simulink model "UltraMaxProPlus"  (R2021a)
settings: Solver=VariableStepAuto  StartTime=0.0  StopTime=2  RelTol=1e-3
undefined symbols (not defined in the file): Ion, Lithium
libraries: spsVoltageMeasurementLib x10, spsCurrentMeasurementLib x8, spsDiodeLib x8, spsSeriesRLCBranchLib x8, spsMeanLib x4, spsMosfetLib x4, spsPowerLib x2, spspowerguiLib x2, spsACVoltageSourceLib x1, spsBatteryLib x1, spsMutualInductanceLib x1, simulink x1
settings Model: SimulationMode=accelerator  Creator=Nishith  LastModifiedBy=Nishith
settings SolverCC: AlgebraicLoopSolver=TrustRegion
settings DebuggingCC: UnconnectedInputMsg=none  UnconnectedOutputMsg=none  UnconnectedLineMsg=none  ArithmeticOperatorsInVariantConditions=warning
settings SFSimCC: CustomCodeUndefinedFunction=UseInterfaceOnly

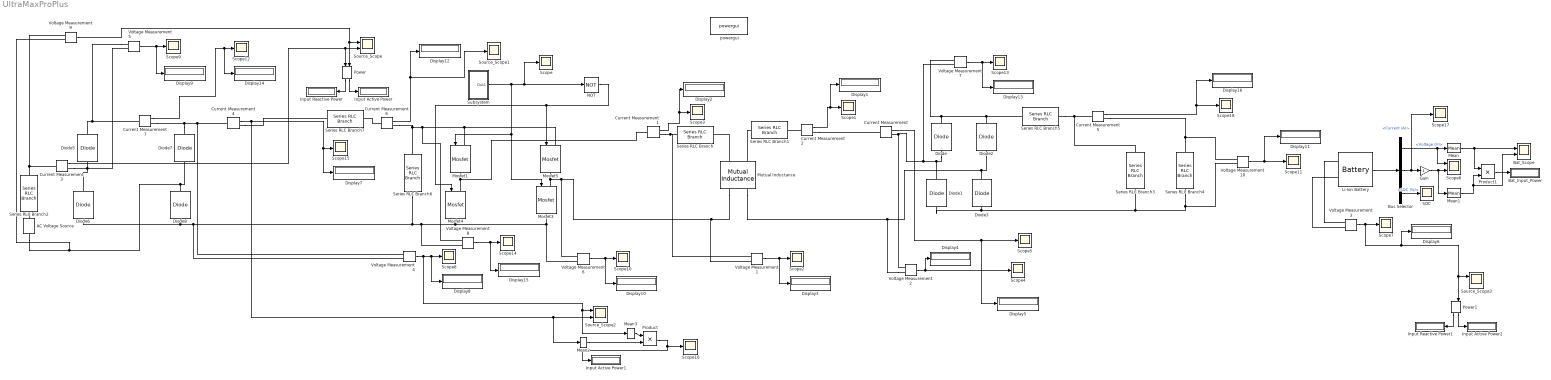
== system UltraMaxProPlus ==
  AC Voltage Source : spsACVoltageSourceLib/AC Voltage Source  Amplitude=325  Phase=0  Frequency=50  SampleTime=0  Measurements=None  BusType=swing  Pref=10e3  Qref=0  Qmin=-inf  Qmax=+inf
  Bat_Input_Power : Display
  Bat_Scope : Scope  NumInputPorts=2
  Bus Selector : BusSelector  OutputSignals=Voltage (V),Current (A),SOC (%)
  Current Measurement{,1..7} (8 alike) : spsCurrentMeasurementLib/Current Measurement  PhasorSimulation=off  OutputType=Complex  PSBequivalent=0
  Diode{,1..3,5..8} (8 alike) : spsDiodeLib/Diode  Ron=0.001  Lon=0  Vf=0.8  IC=0  UseSnubber=0  Rs=500  Cs=250e-9  Measurements=off
  Display{1..16} (16 alike) : Display
  Gain : Gain  Gain=-1
  Input Active Power : Display
  Input Active Power1 : Display
  Input Active Power2 : Display
  Input Reactive Power : Display
  Input Reactive Power1 : Display
  Li-Ion Battery : spsBatteryLib/Battery  BatType=Lithium-Ion  ShowTempParam=off  ThermalPreset=no  ShowAgeParam=off  NomV=120  NomQ=30  SOC=50  Batt_Tr=1  PresetModel=on  MaxQ=30  MinV=90  FullV=139.6785  Dis_rate=13.0435  R=0.04  Normal_OP=27.1304  expZone="[129.6463      1.473913]"  current=[6.5 13 32.5]  Units=Time  Tci=20  NomT=20  T2=-30  MaxQ2=4.8  FullV2=7.1  Normal_OP2=5.655  expZone2="[6.58           1]"  Rca=0.6  ti=2000  Dp=0  Neq0=0  Tsim=1e6  Ta1=25  Qeol=5.4*0.9  Reol=0.013333*1.2  Char_age=[2.3478, 3]  Dis_age=[2.3478, 10]  N1=1500  N2=10500  N3=1000  N4=1400  Ta2=45  N5=950
  Mean : spsMeanLib/Mean  Freq=50  Vinit=0  Ts=0
  Mean1 : spsMeanLib/Mean  Freq=50  Vinit=0  Ts=0
  Mean2 : spsMeanLib/Mean  Freq=60  Vinit=0  Ts=0
  Mean3 : spsMeanLib/Mean  Freq=60  Vinit=0  Ts=0
  Mosfet{1,3..5} (4 alike) : spsMosfetLib/Mosfet  Ron=0.1  Lon=0  Rd=0.01  Vfd=0  IC=0  Rs=1e5  Cs=inf  Measurements=off
  Mutual Inductance : spsMutualInductanceLib/Mutual Inductance  LConnTagsString=a|b  RConnTagsString=A|B  TypeOfMutual=Two or three windings with equal mutual terms  NumberOfWindings=3  SelfImpedance1=[0.001 996.44e-06]  SelfImpedance2=[0.001 107.85e-06]  ThreeWindings=off  SelfImpedance3=[ 1.1 1.1e-03]  MutualImpedance=[0.002 65.5649e-06]  InductanceMatrix="[1.0 0.9  0.9 ;  0.9 1.0  0.9;  0.9 0.9 1.0 ] * 1e-3"  ResistanceMatrix="[1.0 0.9  0.9 ;  0.9 1.0  0.9;  0.9 0.9 1.0 ]"  Measurements=Winding voltages and currents
      settings: SourceProductBaseCode=PS
  NOT : Logic  Operator=NOT  IconShape=distinctive  AllPortsSameDT=off  OutDataTypeStr=boolean
  Power : spsPowerLib/Power  Freq=50  Vinit=[1, 0]  Iinit=[1, 0]  Ts=0
      settings: SourceProductBaseCode=PS
  Power1 : spsPowerLib/Power  Freq=50  Vinit=[1, 0]  Iinit=[1, 0]  Ts=0
      settings: SourceProductBaseCode=PS
  Product : Product
  Product1 : Product
  SOC : Scope
  Scope{,1..5,7..18} (18 alike) : Scope
  Scope6 : Scope  NumInputPorts=2
  Series RLC Branch : spsSeriesRLCBranchLib/Series RLC Branch  LConnTagsString=__new0  RConnTagsString=__new0  BranchType=C  Resistance=1  Inductance=1e-3  SetiL0=off  InitialCurrent=0  Capacitance=3.5184e-9  Setx0=off  InitialVoltage=0  Measurements=None
  Series RLC Branch1 : spsSeriesRLCBranchLib/Series RLC Branch  LConnTagsString=__new0  RConnTagsString=__new0  BranchType=C  Resistance=1  Inductance=1e-3  SetiL0=off  InitialCurrent=0  Capacitance=32.507e-9  Setx0=off  InitialVoltage=0  Measurements=None
  Series RLC Branch2 : spsSeriesRLCBranchLib/Series RLC Branch  LConnTagsString=__new0  RConnTagsString=__new0  BranchType=RL  Resistance=0.1  Inductance=3e-3  SetiL0=off  InitialCurrent=0  Capacitance=1e-6  Setx0=off  InitialVoltage=0  Measurements=None
  Series RLC Branch3 : spsSeriesRLCBranchLib/Series RLC Branch  LConnTagsString=__new0  RConnTagsString=__new0  BranchType=C  Resistance=1  Inductance=1e-3  SetiL0=off  InitialCurrent=0  Capacitance=300e-6  Setx0=off  InitialVoltage=0  Measurements=None
  Series RLC Branch4 : spsSeriesRLCBranchLib/Series RLC Branch  LConnTagsString=__new0  RConnTagsString=__new0  BranchType=R  Resistance=28.8  Inductance=1e-3  SetiL0=off  InitialCurrent=0  Capacitance=1e-6  Setx0=off  InitialVoltage=0  Measurements=None
  Series RLC Branch5 : spsSeriesRLCBranchLib/Series RLC Branch  LConnTagsString=__new0  RConnTagsString=__new0  BranchType=L  Resistance=1  Inductance=5e-3  SetiL0=off  InitialCurrent=0  Capacitance=1e-6  Setx0=off  InitialVoltage=0  Measurements=None
  Series RLC Branch6 : spsSeriesRLCBranchLib/Series RLC Branch  LConnTagsString=__new0  RConnTagsString=__new0  BranchType=C  Resistance=1  Inductance=1e-3  SetiL0=off  InitialCurrent=0  Capacitance=500e-6  Setx0=off  InitialVoltage=0  Measurements=None
  Series RLC Branch7 : spsSeriesRLCBranchLib/Series RLC Branch  LConnTagsString=__new0  RConnTagsString=__new0  BranchType=L  Resistance=1  Inductance=10e-3  SetiL0=off  InitialCurrent=0  Capacitance=1e-6  Setx0=off  InitialVoltage=0  Measurements=None
  Source_Scope : Scope  NumInputPorts=2
  Source_Scope1 : Scope
  Source_Scope2 : Scope  NumInputPorts=2
  Source_Scope3 : Scope  NumInputPorts=2
  Subsystem : Subsystem
  Voltage Measurement{1..10} (10 alike) : spsVoltageMeasurementLib/Voltage Measurement  PhasorSimulation=off  OutputType=Complex  PSBequivalent=0
  powergui : spspowerguiLib/powergui  Priority=1  SimulationMode=Continuous  SampleTime=1e-9  frequency=60  Iterations=50  frequencyindice=0  Pbase=100e6  ErrMax=1e-4  UnitsV=kV  UnitsW=MW  buscounter=0  FunctionMessages=off  echomessages=off  EnableUseOfTLC=off  CurrentSourceSwitches=off  DisableSnubberDevices=off  DisableRonSwitches=off  DisableVfSwitches=off  DisplayEquations=off  AutomaticDiscreteSolvers=off  SolverType=Tustin/Backward Euler (TBE)  Interpol=off  ExternalGateDelay=off  methode=off  Ts=100  x0status=blocks  SPID=on  SwTol=0  HookPort=off  NonlinearTolerance=1e-4  nMaxIteration=100  ContinueOnMaxIteration=off  RestoreLinks=warning  ResistiveCurrentMeasurement=off  Frange=[0:2:500]  Ylog=off  Xlog=on  ShowGrid=off  save=off  variable=ZData  structure=0  ZoomFFT=off  StartTime=0.0  cycles=1  DisplayStyle=1  fundamental=60  FreqAxis=off  MaxFrequency=1000  frequencyindicesteady=1  RmsSteady=1  display=off
  wires:
  Li-Ion Battery/1 -> Bus Selector/1
  Product1/1 -> Bat_Input_Power/1
  Voltage Measurement2/1 -> Display4/1, Scope4/1
  Mean1/1 -> Bat_Scope/2, Product1/2
  Mean/1 -> Bat_Scope/1, Product1/1
  Bus Selector/3 -> SOC/1  "<SOC (%)>"
  Voltage Measurement6/1 -> Display10/1, Scope10/1
  Bus Selector/1 -> Scope6/1, Mean/1  "<Voltage (V)>"
  Current Measurement1/1 -> Display2/1, Scope3/1
  Gain/1 -> Mean1/1, Scope6/2
  Current Measurement6/1 -> Source_Scope1/1, Display12/1
  Current Measurement2/1 -> Display1/1, Scope1/1
  Current Measurement/1 -> Display5/1, Scope5/1
  Voltage Measurement7/1 -> Display13/1, Scope13/1
  Voltage Measurement8/1 -> Display15/1, Scope14/1
  Voltage Measurement5/1 -> Display9/1, Scope9/1
  Subsystem/1(Out1) -> Mosfet3/1, Mosfet1/1, Scope/1, NOT/1
  Current Measurement7/1 -> Display14/1, Scope12/1
  Bus Selector/2 -> Scope17/1, Gain/1  "<Current (A)>"
  NOT/1 -> Mosfet5/1, Mosfet4/1
  Voltage Measurement1/1 -> Display3/1, Scope2/1
  Power/2 -> Input Reactive Power/1
  Current Measurement3/1 -> Power/2, Source_Scope/2
  Power/1 -> Input Active Power/1
  Voltage Measurement9/1 -> Source_Scope/1, Power/1
  Current Measurement4/1 -> Mean2/1, Source_Scope2/2, Display7/1, Scope15/1
  Product/1 -> Scope16/1, Input Active Power1/1
  Voltage Measurement4/1 -> Mean3/1, Source_Scope2/1, Display8/1, Scope8/1
  Mean2/1 -> Product/2
  Mean3/1 -> Product/1
  Power1/1 -> Input Active Power2/1
  Voltage Measurement3/1 -> Source_Scope3/1, Power1/1, Display6/1, Scope7/1
  Power1/2 -> Input Reactive Power1/1
  Voltage Measurement10/1 -> Scope11/1, Display11/1
  Current Measurement5/1 -> Scope18/1, Display16/1
  connections:
  Diode8/LConn1 -- Diode6/LConn1 -- Voltage Measurement4/LConn2 -- Series RLC Branch6/RConn1 -- Voltage Measurement8/LConn2 -- Mosfet3/RConn1 -- Voltage Measurement6/LConn2 -- Mosfet4/RConn1
  Diode3/LConn1 -- Diode1/LConn1 -- Voltage Measurement10/LConn2 -- Series RLC Branch4/RConn1 -- Series RLC Branch3/RConn1
  Mutual Inductance/RConn1 -- Voltage Measurement1/LConn2 -- Mosfet3/LConn1 -- Mosfet5/RConn1 -- Voltage Measurement6/LConn1
  AC Voltage Source/LConn1 -- Voltage Measurement9/LConn2 -- Diode7/LConn1 -- Diode8/RConn1
  Voltage Measurement2/LConn2 -- Mutual Inductance/RConn2 -- Diode2/LConn1 -- Diode3/RConn1
  Mosfet1/LConn1 -- Mosfet5/LConn1 -- Voltage Measurement8/LConn1 -- Series RLC Branch6/LConn1 -- Current Measurement6/RConn1
  Current Measurement1/RConn1 -- Series RLC Branch/LConn1 -- Voltage Measurement1/LConn1
  Li-Ion Battery/LConn1 -- Voltage Measurement3/LConn1
  Mosfet1/RConn1 -- Mosfet4/LConn1 -- Current Measurement1/LConn1
  Diode7/RConn1 -- Current Measurement4/LConn1 -- Voltage Measurement4/LConn1 -- Current Measurement7/RConn1
  Diode5/LConn1 -- Voltage Measurement5/LConn2 -- Current Measurement3/RConn1 -- Diode6/RConn1
  Voltage Measurement7/LConn2 -- Voltage Measurement2/LConn1 -- Current Measurement/RConn1 -- Diode/LConn1 -- Diode1/RConn1
  Voltage Measurement5/LConn1 -- Diode5/RConn1 -- Current Measurement7/LConn1
  Mutual Inductance/LConn2 -- Series RLC Branch1/LConn1
  Voltage Measurement7/LConn1 -- Series RLC Branch5/LConn1 -- Diode2/RConn1 -- Diode/RConn1
  Current Measurement2/RConn1 -- Current Measurement/LConn1
  Mutual Inductance/LConn1 -- Series RLC Branch/RConn1
  Current Measurement2/LConn1 -- Series RLC Branch1/RConn1
  Current Measurement6/LConn1 -- Series RLC Branch7/RConn1
  Current Measurement3/LConn1 -- Voltage Measurement9/LConn1 -- Series RLC Branch2/LConn1
  Current Measurement4/RConn1 -- Series RLC Branch7/LConn1
  Series RLC Branch2/RConn1 -- AC Voltage Source/RConn1
  Current Measurement5/RConn1 -- Voltage Measurement10/LConn1 -- Series RLC Branch4/LConn1
  Voltage Measurement3/LConn2 -- Li-Ion Battery/LConn2
  Series RLC Branch3/LConn1 -- Current Measurement5/LConn1 -- Series RLC Branch5/RConn1

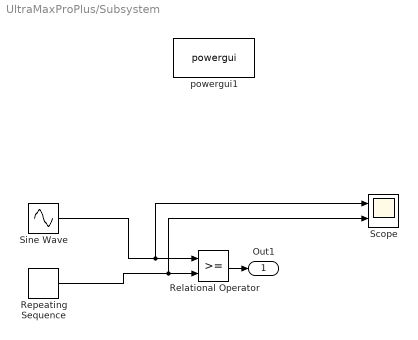
== system UltraMaxProPlus/Subsystem ==
  Relational Operator : RelationalOperator  OutDataTypeStr=boolean  RndMeth=Simplest
  Repeating Sequence : simulink/Sources/Repeating Sequence  rep_seq_t=[0 0.25 0.5 0.75 1]/85000  rep_seq_y=[-1 0 1 0 -1 ]
  Scope : Scope  NumInputPorts=2
  Sine Wave : Sin  Amplitude=0.80  Frequency=2*pi*50  SampleTime=0
  powergui1 : spspowerguiLib/powergui  Priority=1  SimulationMode=Discrete  SampleTime=1e-8  frequency=60  Iterations=50  frequencyindice=0  Pbase=100e6  ErrMax=1e-4  UnitsV=kV  UnitsW=MW  buscounter=0  FunctionMessages=off  echomessages=off  EnableUseOfTLC=off  CurrentSourceSwitches=off  DisableSnubberDevices=off  DisableRonSwitches=off  DisableVfSwitches=off  DisplayEquations=off  AutomaticDiscreteSolvers=off  SolverType=Tustin/Backward Euler (TBE)  Interpol=off  ExternalGateDelay=off  methode=off  Ts=100  x0status=blocks  SPID=on  SwTol=0  HookPort=off  NonlinearTolerance=1e-4  nMaxIteration=100  ContinueOnMaxIteration=off  RestoreLinks=warning  ResistiveCurrentMeasurement=off  Frange=[0:2:500]  Ylog=off  Xlog=on  ShowGrid=off  save=off  variable=ZData  structure=0  ZoomFFT=off  StartTime=0.0  cycles=1  DisplayStyle=1  fundamental=60  FreqAxis=off  MaxFrequency=1000  frequencyindicesteady=1  RmsSteady=1  display=off
  Out1 : Outport
  wires:
  Repeating Sequence/1 -> Scope/2, Relational Operator/2
  Relational Operator/1 -> Out1/1
  Sine Wave/1 -> Scope/1, Relational Operator/1
